simulink model "ESTS_LSM_test"  (R2023b)
settings: Solver=VariableStepAuto  StartTime=0.0  StopTime=10.0  RelTol=1e-3
libraries: ESTS_LSM x1, simulink x1
settings Model: Creator=blatak  LastModifiedBy=blatak

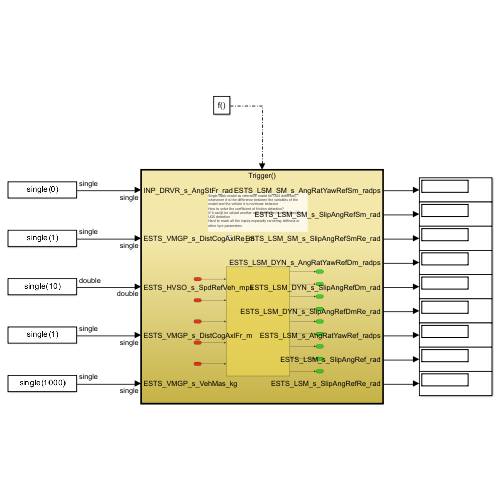
[thumbnail: Simulink's stored preview of the top-level diagram]
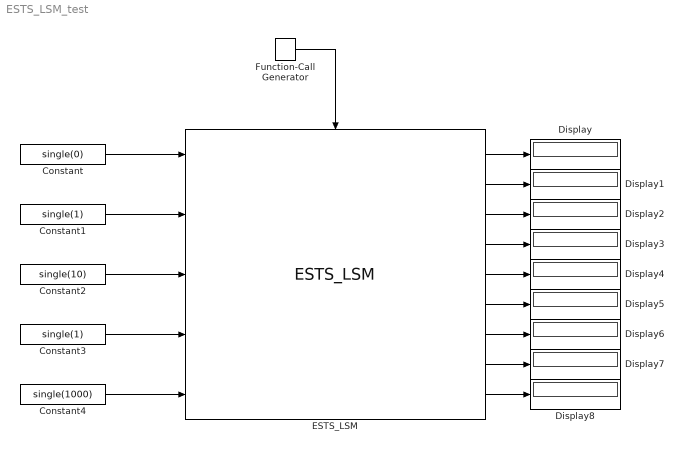
== system ESTS_LSM_test ==
  Constant : Constant  Value=single(0)
  Constant1 : Constant  Value=single(1)
  Constant2 : Constant  Value=single(10)
  Constant3 : Constant  Value=single(1)
  Constant4 : Constant  Value=single(1000)
  Display{,1..8} (9 alike) : Display
  ESTS_LSM : ESTS_LSM/ESTS_LSM  SystemSampleTime=-1  VariantActivationTime=update diagram  AllowFlexibleInterface=on  Latency=0  AutoFrameSizeCalculation=off
      link override ESTS_LSM/Constant1: Value=ESTS_LSM_c_TiSample_s
  Function-Call Generator : simulink/Ports & Subsystems/Function-Call Generator  sample_time=0.01  numberOfIterations=1  DisallowWideOutput=off
  wires:
  Constant/1 -> ESTS_LSM/1
  Constant1/1 -> ESTS_LSM/2
  Constant2/1 -> ESTS_LSM/3
  Constant3/1 -> ESTS_LSM/4
  Constant4/1 -> ESTS_LSM/5
  ESTS_LSM/1 -> Display/1
  ESTS_LSM/2 -> Display1/1
  ESTS_LSM/3 -> Display2/1
  ESTS_LSM/4 -> Display3/1
  ESTS_LSM/5 -> Display4/1
  ESTS_LSM/6 -> Display5/1
  ESTS_LSM/7 -> Display6/1
  ESTS_LSM/8 -> Display7/1
  ESTS_LSM/9 -> Display8/1
  Function-Call Generator/1 -> ESTS_LSM/Trigger
